simulink model "discreteTimeModelP"  (R2014b)
settings: Solver=ode4  StartTime=0.0  StopTime=TIME_SIM  FixedStep=STEP_SIZE  RelTol=1e-3
values from neighbouring files (symbols this model uses):
  C = [1 0 0]    [mainbis.m]
  K = acker(F,G,P)    [mainbis.m]
  Ts = 0.0001    [mainbis.m]
undefined symbols (not defined in the file or in its folder): F, G, Gd
settings Model: Creator=Kate  LastModifiedBy=titou
settings DataIOCC: SaveState=on

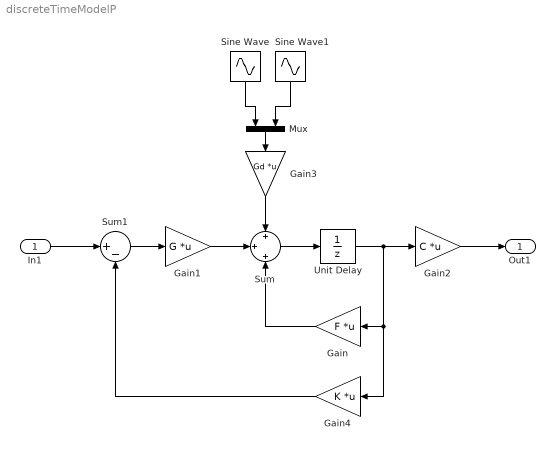
== system discreteTimeModelP ==
  In1 : Inport
  Gain : Gain  Gain=F  Multiplication=Matrix(K*u)
  Gain1 : Gain  Gain=G  Multiplication=Matrix(K*u)
  Gain2 : Gain  Gain=C  Multiplication=Matrix(K*u)
  Gain3 : Gain  Gain=Gd  Multiplication=Matrix(K*u)
  Gain4 : Gain  Gain=K  Multiplication=Matrix(K*u)
  Mux : Mux  Inputs=2
  Sine Wave : Sin  Amplitude=0.0830  Frequency=40  SampleTime=Ts
  Sine Wave1 : Sin  Amplitude=0.0303  Frequency=60  SampleTime=Ts
  Sum : Sum  Inputs=+|+|+
  Sum1 : Sum  Inputs=|+-
  Unit Delay : UnitDelay  SampleTime=Ts
  Out1 : Outport
  wires:
  Sum/1 -> Unit Delay/1
  Unit Delay/1 -> Gain2/1, Gain4/1, Gain/1
  Gain/1 -> Sum/3
  Gain1/1 -> Sum/2
  Gain2/1 -> Out1/1
  Gain3/1 -> Sum/1
  Mux/1 -> Gain3/1
  Sine Wave/1 -> Mux/1
  Sine Wave1/1 -> Mux/2
  In1/1 -> Sum1/1
  Sum1/1 -> Gain1/1
  Gain4/1 -> Sum1/2
